simulink model "sampleModel1984"  (R2023a)
settings: Solver=VariableStepAuto  StartTime=0.0  StopTime=10.0  RelTol=1e-3
libraries: simulink x8, hdlsllib x5
settings Model: Creator=user1  LastModifiedBy=user1

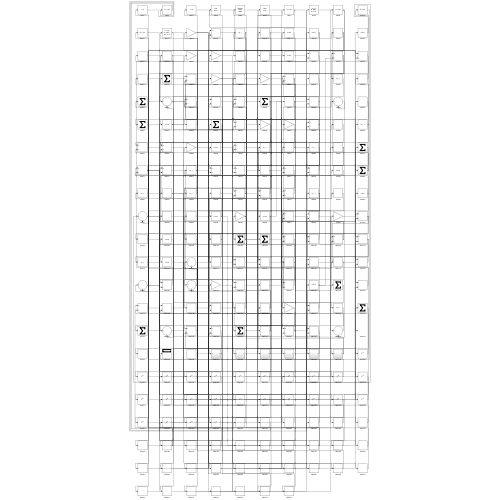
[thumbnail: Simulink's stored preview of the top-level diagram]
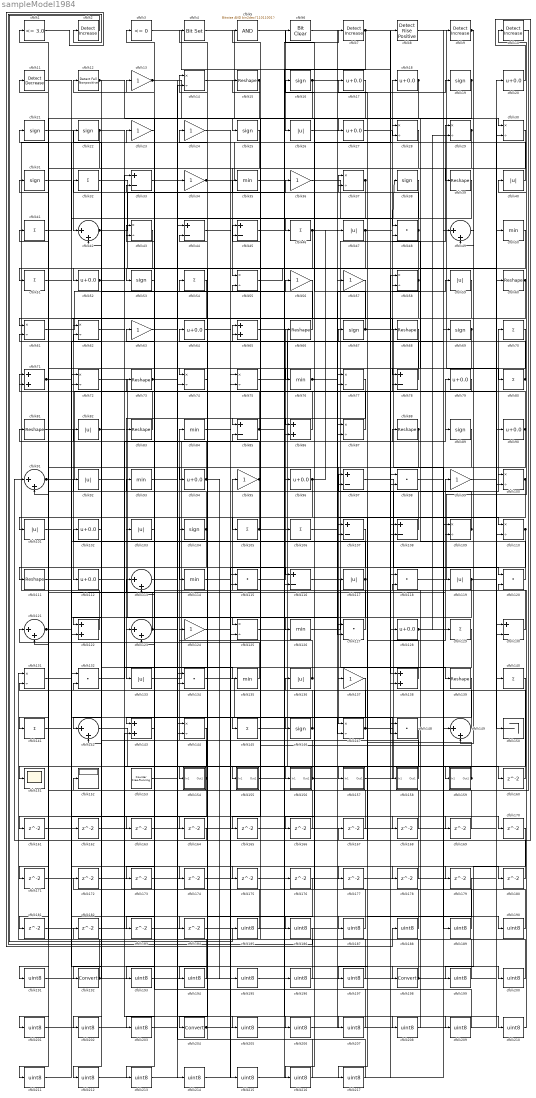
== system sampleModel1984 ==
  cfblk1 : hdlsllib/Logic and Bit Operations/Compare To Constant  relop=<=  const=3.0  OutDataTypeStr=boolean
  cfblk{2,7,9..10} (4 alike) : simulink/Logic and Bit Operations/Detect Increase  vinit=0.0  OutDataTypeStr=boolean
      settings: LibrarySourceBlock=|
      | hdlsllib/Logic and Bit
      | Operations/Detect
      | Increase
  cfblk{14,28..30,37,43,55,58,61..62,72,74..75,77,87,100,109..110,125,131,144,147} (22 alike) : Product  Inputs=*/  RndMeth=Zero  SaturateOnIntegerOverflow=on
  cfblk{26,40,47,59,82,92,101,103,117,119,133,136} (12 alike) : Abs  SaturateOnIntegerOverflow=off
  cfblk{17..18,20,27,52,64,79,90,94,96,102,112,128} (13 alike) : Bias  Bias=0.0  SaturateOnIntegerOverflow=off
  cfblk{16,19,21..22,25,31,38,53,67,69,89,104,146} (13 alike) : Signum
  cfblk{32,41,46,51,54,70,80,105..106,129,140..141,145} (13 alike) : Sum  Inputs=+
  cfblk{33,44..45,78,85,97,107..108,116,130} (10 alike) : Sum  Inputs=+-
  cfblk11 : simulink/Logic and Bit Operations/Detect Decrease  vinit=0.0  OutDataTypeStr=boolean
      settings: LibrarySourceBlock=|
      | hdlsllib/Logic and Bit
      | Operations/Detect
      | Decrease
  cfblk{15,39,60,66,68,73,81,83,88,111,139} (11 alike) : Reshape
  cfblk{42,49,91,113,121,123,142,149} (8 alike) : Sum  Inputs=|++
  cfblk{35,50,76,84,93,114,126,135} (8 alike) : MinMax
  cfblk{48,98,115,118,120,127,132,134,148} (9 alike) : DotProduct  OutDataTypeStr=Inherit: Inherit via internal rule
  cfblk12 : hdlsllib/Logic and Bit Operations/Detect Fall Nonpositive  vinit=0  OutDataTypeStr=boolean
  cfblk{65,71,86,122,138,143} (6 alike) : Sum
  cfblk{13,23..24,34,36,56..57,63,95,99,124,137} (12 alike) : Gain
  cfblk150 : Terminator
  cfblk151 : Scope
  cfblk152 : Display
  cfblk153 : hdlsllib/Sources/Counter Free-Running  NumBits=16  tsamp=-1
  cfblk154 : Subsystem
      settings: LibrarySourceBlock=|
      | hdlsllib/Ports &
      | Subsystems/Subsystem
  cfblk155 : Subsystem
      settings: LibrarySourceBlock=|
      | hdlsllib/Ports &
      | Subsystems/Subsystem
  cfblk156 : Subsystem
      settings: LibrarySourceBlock=|
      | hdlsllib/Ports &
      | Subsystems/Subsystem
  cfblk157 : Subsystem
      settings: LibrarySourceBlock=|
      | hdlsllib/Ports &
      | Subsystems/Subsystem
  cfblk158 : Subsystem
      settings: LibrarySourceBlock=|
      | hdlsllib/Ports &
      | Subsystems/Subsystem
  cfblk159 : Subsystem
      settings: LibrarySourceBlock=|
      | hdlsllib/Ports &
      | Subsystems/Subsystem
  cfblk{160..184} (25 alike) : Delay  SampleTime=1
  cfblk{185..191,193..197,199..203,205..217} (30 alike) : DataTypeConversion  OutDataTypeStr=uint8  SaturateOnIntegerOverflow=off  RndMeth=Floor
  cfblk192 : DataTypeConversion  SaturateOnIntegerOverflow=off  RndMeth=Floor
  cfblk198 : DataTypeConversion  SaturateOnIntegerOverflow=off  RndMeth=Floor
  cfblk204 : DataTypeConversion  SaturateOnIntegerOverflow=off  RndMeth=Floor
  cfblk3 : hdlsllib/Logic and Bit Operations/Compare To Zero  relop=<=  OutDataTypeStr=boolean
  cfblk4 : simulink/Logic and Bit Operations/Bit Set  iBit=0
      settings: LibrarySourceBlock=|
      | hdlsllib/Logic and Bit
      | Operations/Bit Set
  cfblk5 : simulink/Logic and Bit Operations/Bitwise Operator  logicop=AND  UseBitMask=on  BitMask=bin2dec('11011001')  BitMaskRealWorld=Stored Integer
      settings: LibrarySourceBlock=|
      | hdlsllib/Logic and Bit
      | Operations/Bitwise
      | Operator
  cfblk6 : simulink/Logic and Bit Operations/Bit Clear  iBit=0
      settings: LibrarySourceBlock=|
      | hdlsllib/Logic and Bit
      | Operations/Bit Clear
  cfblk8 : hdlsllib/Logic and Bit Operations/Detect Rise Positive  vinit=0  OutDataTypeStr=boolean
  wires:
  cfblk61/1 -> cfblk56/1
  cfblk125/1 -> cfblk159/1(In1)
  cfblk96/1 -> cfblk47/1, cfblk181/1
  cfblk122/1 -> cfblk23/1
  cfblk102/1 -> cfblk142/1
  cfblk154/1(Out1) -> cfblk84/1, cfblk161/1
  cfblk4/1 -> cfblk27/1
  cfblk53/1 -> cfblk12/1
  cfblk55/1 -> cfblk133/1
  cfblk105/1 -> cfblk101/1, cfblk19/1, cfblk170/1
  cfblk88/1 -> cfblk147/1, cfblk91/2
  cfblk85/1 -> cfblk43/2, cfblk207/1
  cfblk133/1 -> cfblk79/1
  cfblk65/1 -> cfblk147/2
  cfblk147/1 -> cfblk70/1, cfblk85/2
  cfblk13/1 -> cfblk25/1, cfblk48/1, cfblk155/1(In1)
  cfblk62/1 -> cfblk154/1(In1)
  cfblk54/1 -> cfblk112/1
  cfblk118/1 -> cfblk10/1
  cfblk42/1 -> cfblk36/1, cfblk150/1
  cfblk90/1 -> cfblk18/1, cfblk203/1
  cfblk115/1 -> cfblk66/1
  cfblk72/1 -> cfblk125/1
  cfblk127/1 -> cfblk95/1
  cfblk119/1 -> cfblk60/1, cfblk173/1
  cfblk97/1 -> cfblk120/1
  cfblk47/1 -> cfblk38/1, cfblk74/2, cfblk104/1
  cfblk8/1 -> cfblk80/1
  cfblk139/1 -> cfblk145/1
  cfblk116/1 -> cfblk139/1
  cfblk57/1 -> cfblk123/1
  cfblk117/1 -> cfblk156/1(In1), cfblk42/2
  cfblk59/1 -> cfblk83/1
  cfblk132/1 -> cfblk89/1
  cfblk21/1 -> cfblk42/1
  cfblk136/1 -> cfblk14/1, cfblk65/2
  cfblk58/1 -> cfblk52/1, cfblk75/2
  cfblk77/1 -> cfblk103/1
  cfblk76/1 -> cfblk59/1, cfblk216/1
  cfblk15/1 -> cfblk53/1, cfblk134/2
  cfblk126/1 -> cfblk29/1
  cfblk104/1 -> cfblk71/1, cfblk123/2
  cfblk79/1 -> cfblk71/2
  cfblk38/1 -> cfblk46/1
  cfblk75/1 -> cfblk9/1
  cfblk91/1 -> cfblk49/1, cfblk200/1
  cfblk157/1(Out1) -> cfblk99/1
  cfblk66/1 -> cfblk22/1
  cfblk10/1 -> cfblk152/1
  cfblk56/1 -> cfblk62/1
  cfblk69/1 -> cfblk111/1, cfblk115/2
  cfblk12/1 -> cfblk122/1, cfblk30/2
  cfblk3/1 -> cfblk138/1
  cfblk50/1 -> cfblk204/1
  cfblk142/1 -> cfblk157/1(In1)
  cfblk19/1 -> cfblk78/1, cfblk165/1
  cfblk103/1 -> cfblk143/1
  cfblk134/1 -> cfblk158/1(In1)
  cfblk141/1 -> cfblk119/1
  cfblk28/1 -> cfblk122/2
  cfblk25/1 -> cfblk55/1
  cfblk48/1 -> cfblk32/1, cfblk146/1
  cfblk140/1 -> cfblk192/1
  cfblk158/1(Out1) -> cfblk54/1
  cfblk121/1 -> cfblk67/1, cfblk169/1
  cfblk22/1 -> cfblk51/1, cfblk174/1
  cfblk46/1 -> cfblk74/1, cfblk110/1
  cfblk87/1 -> cfblk45/1
  cfblk109/1 -> cfblk24/1, cfblk48/2
  cfblk108/1 -> cfblk17/1
  cfblk89/1 -> cfblk94/1
  cfblk80/1 -> cfblk64/1, cfblk65/1
  cfblk128/1 -> cfblk69/1, cfblk29/2
  cfblk159/1(Out1) -> cfblk97/1, cfblk5/1
  cfblk143/1 -> cfblk113/1
  cfblk120/1 -> cfblk58/2
  cfblk146/1 -> cfblk11/1, cfblk43/1
  cfblk110/1 -> cfblk197/1, cfblk213/1
  cfblk156/1(Out1) -> cfblk107/1, cfblk61/2
  cfblk155/1(Out1) -> cfblk7/1
  cfblk29/1 -> cfblk86/1, cfblk105/1
  cfblk135/1 -> cfblk121/1
  cfblk32/1 -> cfblk117/1
  cfblk9/1 -> cfblk39/1, cfblk49/2
  cfblk106/1 -> cfblk100/1
  cfblk99/1 -> cfblk90/1
  cfblk86/1 -> cfblk41/1
  cfblk41/1 -> cfblk28/1
  cfblk39/1 -> cfblk126/1
  cfblk14/1 -> cfblk130/1
  cfblk5/1 -> cfblk26/1
  cfblk37/1 -> cfblk72/2, cfblk142/2
  cfblk95/1 -> cfblk114/1, cfblk82/1
  cfblk78/1 -> cfblk15/1
  cfblk138/1 -> cfblk37/1
  cfblk74/1 -> cfblk4/1
  cfblk27/1 -> cfblk28/2
  cfblk71/1 -> cfblk148/2, cfblk127/2, cfblk177/1
  cfblk131/1 -> cfblk198/1
  cfblk67/1 -> cfblk149/1, cfblk6/1
  cfblk149/1 -> cfblk62/2
  cfblk94/1 -> cfblk31/1, cfblk195/1
  cfblk82/1 -> cfblk179/1, cfblk180/1
  cfblk45/1 -> cfblk106/1
  cfblk83/1 -> cfblk73/1
  cfblk60/1 -> cfblk40/1, cfblk61/1
  cfblk81/1 -> cfblk20/1
  cfblk68/1 -> cfblk141/1
  cfblk145/1 -> cfblk86/2
  cfblk40/1 -> cfblk16/1
  cfblk112/1 -> cfblk135/1
  cfblk26/1 -> cfblk127/1
  cfblk11/1 -> cfblk68/1
  cfblk18/1 -> cfblk76/1, cfblk211/1
  cfblk73/1 -> cfblk13/1, cfblk78/2
  cfblk36/1 -> cfblk108/1
  cfblk24/1 -> cfblk75/1
  cfblk34/1 -> cfblk8/1, cfblk178/1
  cfblk114/1 -> cfblk116/1
  cfblk111/1 -> cfblk109/2
  cfblk113/1 -> cfblk88/1
  cfblk7/1 -> cfblk30/1, cfblk116/2
  cfblk43/1 -> cfblk151/1
  cfblk6/1 -> cfblk57/1
  cfblk49/1 -> cfblk149/2
  cfblk16/1 -> cfblk121/2, cfblk108/2
  cfblk70/1 -> cfblk85/1
  cfblk123/1 -> cfblk81/1, cfblk168/1
  cfblk100/1 -> cfblk137/1, cfblk183/1
  cfblk130/1 -> cfblk3/1
  cfblk52/1 -> cfblk33/1, cfblk55/2
  cfblk84/1 -> cfblk160/1
  cfblk160/1 -> cfblk72/1
  cfblk161/1 -> cfblk130/2
  cfblk23/1 -> cfblk163/1
  cfblk163/1 -> cfblk14/2
  cfblk101/1 -> cfblk164/1
  cfblk164/1 -> cfblk91/1
  cfblk165/1 -> cfblk109/1
  cfblk30/1 -> cfblk166/1
  cfblk166/1 -> cfblk45/2
  cfblk20/1 -> cfblk167/1
  cfblk167/1 -> cfblk1/1
  cfblk168/1 -> cfblk97/2
  cfblk169/1 -> cfblk134/1
  cfblk107/1 -> cfblk171/1
  cfblk171/1 -> cfblk125/2
  cfblk172/1 -> cfblk77/2
  cfblk173/1 -> cfblk110/2
  cfblk174/1 -> cfblk58/1
  cfblk51/1 -> cfblk175/1
  cfblk175/1 -> cfblk100/2
  cfblk177/1 -> cfblk138/2
  cfblk178/1 -> cfblk33/2
  cfblk180/1 -> cfblk37/2
  cfblk181/1 -> cfblk143/2
  cfblk182/1 -> cfblk87/2
  cfblk183/1 -> cfblk113/2
  cfblk92/1 -> cfblk184/1
  cfblk2/1 -> cfblk185/1
  cfblk185/1 -> cfblk92/1
  cfblk184/1 -> cfblk186/1
  cfblk186/1 -> cfblk2/1
  cfblk93/1 -> cfblk187/1
  cfblk187/1 -> cfblk136/1
  cfblk1/1 -> cfblk188/1
  cfblk188/1 -> cfblk93/1
  cfblk98/1 -> cfblk189/1
  cfblk189/1 -> cfblk172/1
  cfblk31/1 -> cfblk190/1
  cfblk190/1 -> cfblk98/1
  cfblk17/1 -> cfblk191/1
  cfblk191/1 -> cfblk98/2
  cfblk192/1 -> cfblk182/1, cfblk21/1, cfblk102/1
  cfblk137/1 -> cfblk193/1
  cfblk193/1 -> cfblk140/1
  cfblk176/1 -> cfblk194/1
  cfblk194/1 -> cfblk132/1
  cfblk195/1 -> cfblk176/1
  cfblk35/1 -> cfblk196/1
  cfblk196/1 -> cfblk132/2
  cfblk197/1 -> cfblk35/1
  cfblk198/1 -> cfblk148/1, cfblk87/1
  cfblk170/1 -> cfblk199/1
  cfblk199/1 -> cfblk131/1
  cfblk200/1 -> cfblk131/2
  cfblk144/1 -> cfblk201/1
  cfblk201/1 -> cfblk34/1
  cfblk148/1 -> cfblk202/1
  cfblk202/1 -> cfblk144/1
  cfblk203/1 -> cfblk144/2
  cfblk204/1 -> cfblk107/2, cfblk77/1
  cfblk33/1 -> cfblk205/1
  cfblk205/1 -> cfblk50/1
  cfblk63/1 -> cfblk206/1
  cfblk206/1 -> cfblk118/1
  cfblk207/1 -> cfblk63/1
  cfblk124/1 -> cfblk208/1
  cfblk208/1 -> cfblk118/2
  cfblk64/1 -> cfblk209/1
  cfblk209/1 -> cfblk124/1
  cfblk162/1 -> cfblk210/1
  cfblk210/1 -> cfblk120/2
  cfblk211/1 -> cfblk162/1
  cfblk129/1 -> cfblk212/1
  cfblk212/1 -> cfblk128/1
  cfblk213/1 -> cfblk129/1
  cfblk153/1 -> cfblk214/1
  cfblk214/1 -> cfblk115/1
  cfblk44/1 -> cfblk215/1
  cfblk215/1 -> cfblk96/1
  cfblk216/1 -> cfblk44/1
  cfblk179/1 -> cfblk217/1
  cfblk217/1 -> cfblk44/2

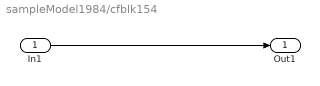
== system sampleModel1984/cfblk154 ==
  In1 : Inport
  Out1 : Outport
  wires:
  In1/1 -> Out1/1

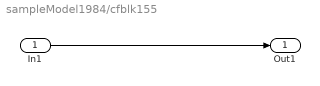
== system sampleModel1984/cfblk155 ==
  In1 : Inport
  Out1 : Outport
  wires:
  In1/1 -> Out1/1

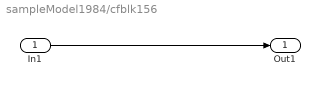
== system sampleModel1984/cfblk156 ==
  In1 : Inport
  Out1 : Outport
  wires:
  In1/1 -> Out1/1

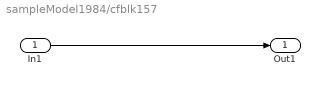
== system sampleModel1984/cfblk157 ==
  In1 : Inport
  Out1 : Outport
  wires:
  In1/1 -> Out1/1

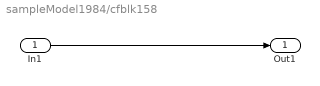
== system sampleModel1984/cfblk158 ==
  In1 : Inport
  Out1 : Outport
  wires:
  In1/1 -> Out1/1

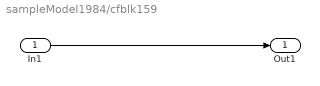
== system sampleModel1984/cfblk159 ==
  In1 : Inport
  Out1 : Outport
  wires:
  In1/1 -> Out1/1
